simulink model "model_double_pendulum"  (R2021b)
settings: Solver=VariableStepAuto  StartTime=0.0  StopTime=10  RelTol=1e-3  EnableMultiTasking=on
InitFcn:
  | m=4;
  | m1=3;
  | m2=1.5;
  | l1=0.5;
  | l2=0.35;
  | g=9.81;
undefined symbols (not defined in the file or in its folder): A, A1_etm4, A1_zv, A2_etm4, A2_zv, A3_etm4, A4_etm4, B, b0, C, D1, Kd, Kp, L, l, L2, t2_etm4, t2_zv, t3_etm4, t4_etm4
settings Model: Creator=ADMIN  LastModifiedBy=Admin
settings DataIOCC: ReturnWorkspaceOutputs=off
settings OptimizationCC: LifeSpan=inf
settings DebuggingCC: SFUnexpectedBacktrackingDiag=warning  SFNoUnconditionalDefaultTransitionDiag=warning  SFMachineParentedDataDiag=warning  ArithmeticOperatorsInVariantConditions=warning
settings SFSimCC: SimUseLocalCustomCode=off  CustomCodeUndefinedFunction=UseInterfaceOnly
settings RTWCC: RTWUseLocalCustomCode=off
settings CodeAppCC: StateflowObjectComments=on
settings GRTTargetCC: TargetLangStandard=C89/C90 (ANSI)
settings ConfigComp: CovMetricSettings=dw  CovSaveCumulativeToWorkspaceVar=on  CovSaveSingleToWorkspaceVar=on  CovExternalEMLEnable=off

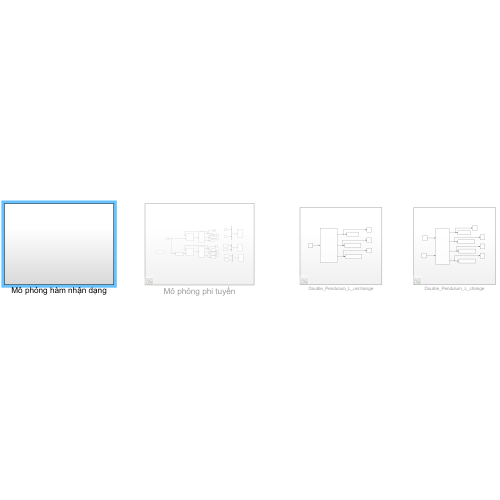
[thumbnail: Simulink's stored preview of the top-level diagram]
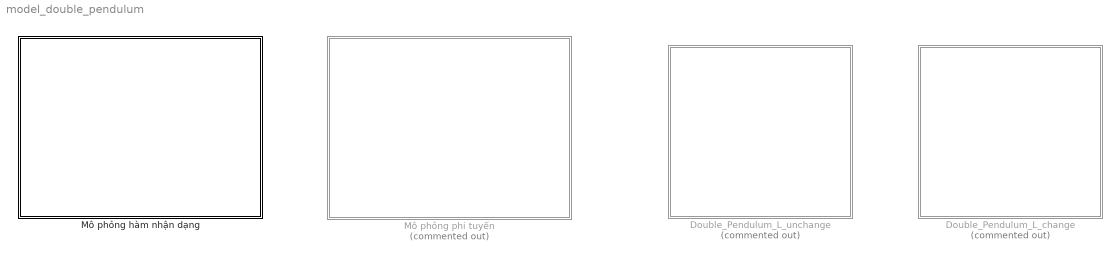
== system model_double_pendulum ==
  Double_Pendulum_L_change : Subsystem  Commented=on
  Double_Pendulum_L_unchange : Subsystem  Commented=on
  Mô phỏng hàm nhận dạng : Subsystem
  Mô phỏng phi tuyến : Subsystem  Commented=on

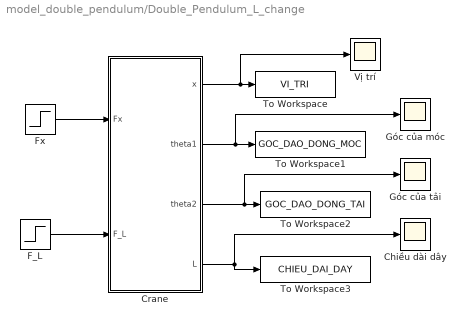
== system model_double_pendulum/Double_Pendulum_L_change ==
  Chiều dài dây : Scope
  "Crane " : Subsystem
  F_L : Step  Time=0  After=10  SampleTime=0
  Fx : Step  Time=0  After=10  SampleTime=0
  Góc của móc : Scope
  Góc của tải : Scope
  To Workspace : ToWorkspace  VariableName=VI_TRI  SaveFormat=Timeseries  SampleTime=-1
  To Workspace1 : ToWorkspace  VariableName=GOC_DAO_DONG_MOC  SaveFormat=Timeseries  SampleTime=-1
  To Workspace2 : ToWorkspace  VariableName=GOC_DAO_DONG_TAI  SaveFormat=Timeseries  SampleTime=-1
  To Workspace3 : ToWorkspace  VariableName=CHIEU_DAI_DAY  SaveFormat=Timeseries  SampleTime=-1
  Vị trí : Scope
  wires:
  Fx/1 -> "Crane "/1("Fx ")
  F_L/1 -> "Crane "/2(F_L)
  "Crane "/1("x ") -> Vị trí/1, To Workspace/1
  "Crane "/3(theta2) -> Góc của tải/1, To Workspace2/1
  "Crane "/4(L) -> To Workspace3/1, Chiều dài dây/1
  "Crane "/2(theta1) -> Góc của móc/1, To Workspace1/1

== system model_double_pendulum/Double_Pendulum_L_unchange ==
  "Crane " : Subsystem
  Fx : Step  Time=0  After=10  SampleTime=0
  Góc của móc : Scope
  Góc của tải : Scope
  To Workspace : ToWorkspace  VariableName=VI_TRI1  SaveFormat=Timeseries  SampleTime=-1
  To Workspace1 : ToWorkspace  VariableName=GOC_DAO_DONG_MOC1  SaveFormat=Timeseries  SampleTime=-1
  To Workspace2 : ToWorkspace  VariableName=GOC_DAO_DONG_TAI1  SaveFormat=Timeseries  SampleTime=-1
  Vị trí : Scope
  wires:
  "Crane "/2(theta1) -> Góc của móc/1, To Workspace1/1
  "Crane "/1("x ") -> Vị trí/1, To Workspace/1
  Fx/1 -> "Crane "/1("Fx ")
  "Crane "/3(theta2) -> Góc của tải/1, To Workspace2/1

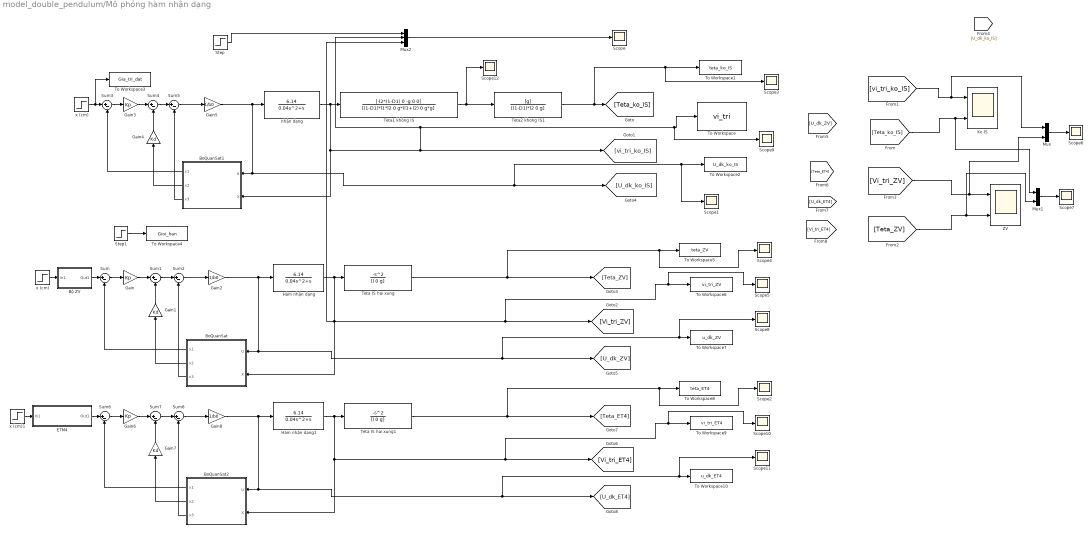
== system model_double_pendulum/Mô phỏng hàm nhận dạng ==
  " nhận dạng" : TransferFcn  Numerator=[6.14]  Denominator="[0.04 1  0]"
  BoQuanSat : Subsystem
  BoQuanSat1 : Subsystem
  BoQuanSat2 : Subsystem
  Bộ ZV : Subsystem
  ETM4 : Subsystem
  Gain : Gain  Gain=Kp
  Gain1 : Gain  Gain=Kd
  Gain2 : Gain  Gain=1/b0
  Gain3 : Gain  Gain=Kp
  Gain4 : Gain  Gain=Kd
  Gain5 : Gain  Gain=1/b0
  Gain6 : Gain  Gain=Kp
  Gain7 : Gain  Gain=Kd
  Gain8 : Gain  Gain=1/b0
  Hàm nhận dạng : TransferFcn  Numerator=[6.14]  Denominator="[0.04 1  0]"
  Hàm nhận dạng1 : TransferFcn  Numerator=[6.14]  Denominator="[0.04 1  0]"
  Ko IS : Scope  NumInputPorts=2
  Mux : Mux  Inputs=2
  Mux1 : Mux  Inputs=2
  Mux2 : Mux  Inputs=3
  Scope{,1..12} (13 alike) : Scope
  Step : Step  Time=0  After=49  SampleTime=0
  Step1 : Step  Time=0  After=10  SampleTime=0
  Sum{,1..8} (9 alike) : Sum  Inputs=|+-
  Teta IS hai xung : TransferFcn  Numerator=[-1 0 0]  Denominator=[l 0 g]
  Teta IS hai xung1 : TransferFcn  Numerator=[-1 0 0]  Denominator=[l 0 g]
  "Teta1 không IS " : TransferFcn  Numerator=[-l2*(1-D1) 0 -g 0 0]  Denominator=[(1-D1)*l1*l2 0 g*(l1+l2) 0 g*g]
  Teta2 khong IS1 : TransferFcn  Numerator=[g]  Denominator=[(1-D1)*l2 0 g]
  To Workspace : ToWorkspace  VariableName=vi_tri  SaveFormat=Timeseries  SampleTime=0.005
  To Workspace1 : ToWorkspace  VariableName=teta_ko_IS  SaveFormat=Timeseries  SampleTime=-1
  To Workspace10 : ToWorkspace  VariableName=u_dk_ET4  SaveFormat=Timeseries  SampleTime=-1
  To Workspace2 : ToWorkspace  VariableName=U_dk_ko_IS  SaveFormat=Timeseries  SampleTime=-1
  To Workspace3 : ToWorkspace  VariableName=Gia_tri_dat  SaveFormat=Timeseries  SampleTime=0.005
  To Workspace4 : ToWorkspace  VariableName=Gioi_han  SaveFormat=Timeseries  SampleTime=-1
  To Workspace5 : ToWorkspace  VariableName=teta_ZV  SaveFormat=Timeseries  SampleTime=-1
  To Workspace6 : ToWorkspace  VariableName=vi_tri_ZV  SaveFormat=Timeseries  SampleTime=-1
  To Workspace7 : ToWorkspace  VariableName=u_dk_ZV  SaveFormat=Timeseries  SampleTime=-1
  To Workspace8 : ToWorkspace  VariableName=teta_ET4  SaveFormat=Timeseries  SampleTime=-1
  To Workspace9 : ToWorkspace  VariableName=vi_tri_ET4  SaveFormat=Timeseries  SampleTime=-1
  ZV : Scope  NumInputPorts=2
  x (cm) : Step  Time=0  After=50  SampleTime=0
  "x (cm) " : Step  Time=0  After=50  SampleTime=0
  x (cm)1 : Step  Time=0  After=50  SampleTime=0
  wires:
  Gain/1 -> Sum1/1
  Sum2/1 -> Gain2/1
  BoQuanSat/2(x2) -> Gain1/1
  BoQuanSat/3(x3) -> Sum2/2
  BoQuanSat/1(x1) -> Sum/2
  Sum/1 -> Gain/1
  Sum1/1 -> Sum2/1
  Gain1/1 -> Sum1/2
  Gain2/1 -> Hàm nhận dạng/1, Scope8/1, To Workspace7/1, [U_dk_ZV], BoQuanSat/1(U)
  x (cm)/1 -> Bộ ZV/1(In1)
  Bộ ZV/1(Out1) -> Sum/1
  Gain4/1 -> Sum4/2
  Sum4/1 -> Sum5/1
  Sum5/1 -> Gain5/1
  BoQuanSat1/1(x1) -> Sum3/2
  BoQuanSat1/3(x3) -> Sum5/2
  BoQuanSat1/2(x2) -> Gain4/1
  Sum3/1 -> Gain3/1
  Gain3/1 -> Sum4/1
  Teta IS hai xung/1 -> Scope4/1, To Workspace5/1, [Teta_ZV]
  [vi_tri_ko_IS] -> Mux/1, Ko IS/1
  [Vi_tri_ZV] -> Mux/2, ZV/1
  [Teta_ZV] -> Mux1/2, ZV/2
  [Teta_ko_IS] -> Mux1/1, Ko IS/2
  Mux/1 -> Scope6/1
  Mux1/1 -> Scope7/1
  " nhận dạng"/1 -> "Teta1 không IS "/1, Scope9/1, To Workspace/1, Mux2/2, [vi_tri_ko_IS], BoQuanSat1/2(X)
  Gain5/1 -> " nhận dạng"/1, Scope1/1, To Workspace2/1, [U_dk_ko_IS], BoQuanSat1/1(U)
  Hàm nhận dạng/1 -> Teta IS hai xung/1, Scope5/1, To Workspace6/1, [Vi_tri_ZV], Mux2/3, BoQuanSat/2(X)
  Step/1 -> Mux2/1
  Mux2/1 -> Scope/1
  "x (cm) "/1 -> To Workspace3/1, Sum3/1
  Step1/1 -> To Workspace4/1
  BoQuanSat2/3(x3) -> Sum8/2
  Teta IS hai xung1/1 -> Scope2/1, To Workspace8/1, [Teta_ET4]
  x (cm)1/1 -> ETM4/1(In1)
  ETM4/1(Out1) -> Sum6/1
  Hàm nhận dạng1/1 -> Teta IS hai xung1/1, Scope10/1, To Workspace9/1, [Vi_tri_ET4], BoQuanSat2/2(X)
  BoQuanSat2/2(x2) -> Gain7/1
  Sum7/1 -> Sum8/1
  BoQuanSat2/1(x1) -> Sum6/2
  Sum6/1 -> Gain6/1
  Sum8/1 -> Gain8/1
  Gain6/1 -> Sum7/1
  Gain8/1 -> Hàm nhận dạng1/1, Scope11/1, To Workspace10/1, [U_dk_ET4], BoQuanSat2/1(U)
  Gain7/1 -> Sum7/2
  "Teta1 không IS "/1 -> Teta2 khong IS1/1, Scope12/1
  Teta2 khong IS1/1 -> Scope3/1, To Workspace1/1, [Teta_ko_IS]

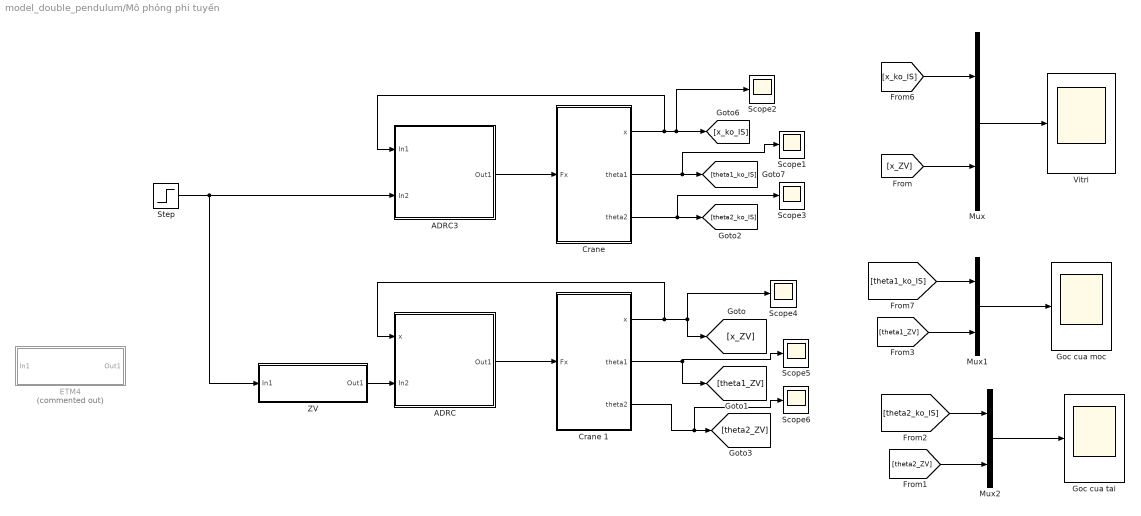
== system model_double_pendulum/Mô phỏng phi tuyến ==
  ADRC : Subsystem
  ADRC3 : Subsystem
  "Crane " : Subsystem
  Crane 1 : Subsystem
  ETM4 : Subsystem  Commented=on
  Goc cua moc : Scope
  Goc cua tai : Scope
  Mux : Mux  Inputs=2
  Mux1 : Mux  Inputs=2
  Mux2 : Mux  Inputs=2
  Scope{1..6} (6 alike) : Scope
  Step : Step  Time=0  After=40  SampleTime=0
  Vitri : Scope
  ZV : Subsystem
  wires:
  [theta1_ko_IS] -> Mux1/1
  Crane 1/1("x ") -> [x_ZV], Scope4/1, ADRC/1("x ")
  Mux1/1 -> Goc cua moc/1
  ADRC/1(Out1) -> Crane 1/1("Fx ")
  Step/1 -> ADRC3/2(In2), ZV/1(In1)
  Mux/1 -> Vitri/1
  [x_ko_IS] -> Mux/1
  "Crane "/1("x ") -> Scope2/1, [x_ko_IS], ADRC3/1(In1)
  ADRC3/1(Out1) -> "Crane "/1("Fx ")
  "Crane "/2(theta1) -> Scope1/1, [theta1_ko_IS]
  ZV/1(Out1) -> ADRC/2(In2)
  [x_ZV] -> Mux/2
  "Crane "/3(theta2) -> Scope3/1, [theta2_ko_IS]
  Crane 1/2(theta1) -> [theta1_ZV], Scope5/1
  [theta1_ZV] -> Mux1/2
  Crane 1/3(theta2) -> Scope6/1, [theta2_ZV]
  [theta2_ZV] -> Mux2/2
  Mux2/1 -> Goc cua tai/1
  [theta2_ko_IS] -> Mux2/1

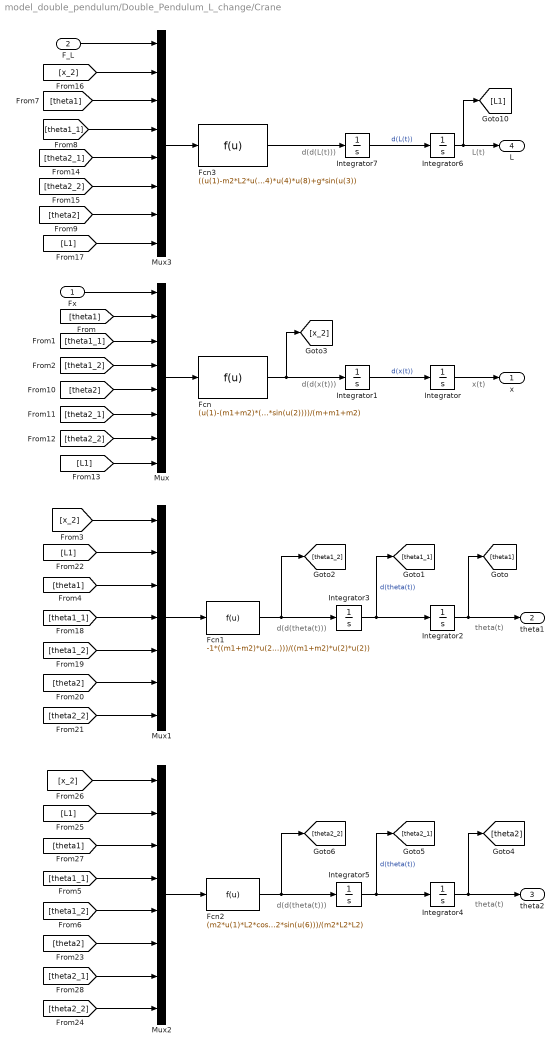
== system model_double_pendulum/Double_Pendulum_L_change/Crane  ==
  note: d(d(x(t)))
  note: x(t)
  note: d(d(theta(t)))
  note: theta(t)
  note: d(d(theta(t)))
  note: theta(t)
  note: L(t)
  note: d(d(L(t)))
  "Fx " : Inport
  F_L : Inport  Port=2
  Fcn : Fcn  Expr=(u(1)-(m1+m2)*(u(4)*u(8)*cos(u(2))-u(3)*u(3)*u(8)*sin(u(2))))/(m+m1+m2)
  Fcn1 : Fcn  Expr=-1*((m1+m2)*u(2)*u(1)*cos(u(3))+m2*u(2)*L2*(u(7)*cos(u(3)-u(6))+u(4)*u(4)*sin(u(3)-u(6)))+(m1+m2)*g*u(2)*sin(u(3)))/((m1+m2)*u(2)*u(2))
  Fcn2 : Fcn  Expr=(m2*u(1)*L2*cos(u(6))+m2*u(2)*L2*u(5)*cos(u(3)-u(6))-m2*u(2)*L2*u(4)*u(4)*sin(u(3)-u(6))+m2*g*L2*sin(u(6)))/(m2*L2*L2)
  Fcn3 : Fcn  Expr=((u(1)-m2*L2*u(6)*sin(u(3)-u(7))+m2*L2*u(5)*u(5)*cos(u(3)-u(7)))/(m1+m2))-u(2)*sin(u(3))+u(4)*u(4)*u(8)+g*sin(u(3))
  Integrator{,1..5,7} (7 alike) : Integrator
  Integrator6 : Integrator  InitialCondition=0.5
  Mux : Mux  Inputs=8
  Mux1 : Mux  Inputs=7
  Mux2 : Mux  Inputs=8
  Mux3 : Mux  Inputs=8
  "x " : Outport
  theta1 : Outport  Port=2
  theta2 : Outport  Port=3
  L : Outport  Port=4
  wires:
  Integrator/1 -> "x "/1
  Integrator1/1 -> Integrator/1  "d(x(t))"
  Integrator2/1 -> [theta1], theta1/1
  Integrator3/1 -> [theta1_1], Integrator2/1  "d(theta(t))"
  Fcn/1 -> [x_2], Integrator1/1
  Mux/1 -> Fcn/1
  "Fx "/1 -> Mux/1
  [theta1] -> Mux/2
  [theta1_1] -> Mux/3
  [theta1_2] -> Mux/4
  Mux1/1 -> Fcn1/1
  Fcn1/1 -> [theta1_2], Integrator3/1
  Mux2/1 -> Fcn2/1
  Fcn2/1 -> [theta2_2], Integrator5/1
  Integrator5/1 -> [theta2_1], Integrator4/1  "d(theta(t))"
  Integrator4/1 -> [theta2], theta2/1
  F_L/1 -> Mux3/1
  Mux3/1 -> Fcn3/1
  Fcn3/1 -> Integrator7/1
  Integrator7/1 -> Integrator6/1  "d(L(t))"
  Integrator6/1 -> [L1], L/1
  [theta2] -> Mux/5
  [theta2_1] -> Mux/6
  [theta2_2] -> Mux/7
  [L1] -> Mux/8
  [theta2_1] -> Mux3/5
  [theta2_2] -> Mux3/6
  [theta1] -> Mux3/3
  [theta1_1] -> Mux3/4
  [x_2] -> Mux3/2
  [theta2] -> Mux3/7
  [L1] -> Mux3/8
  [x_2] -> Mux1/1
  [L1] -> Mux1/2
  [theta1] -> Mux1/3
  [theta1_1] -> Mux1/4
  [theta1_2] -> Mux1/5
  [theta2] -> Mux1/6
  [theta2_2] -> Mux1/7
  [x_2] -> Mux2/1
  [L1] -> Mux2/2
  [theta1] -> Mux2/3
  [theta1_1] -> Mux2/4
  [theta1_2] -> Mux2/5
  [theta2] -> Mux2/6
  [theta2_1] -> Mux2/7
  [theta2_2] -> Mux2/8

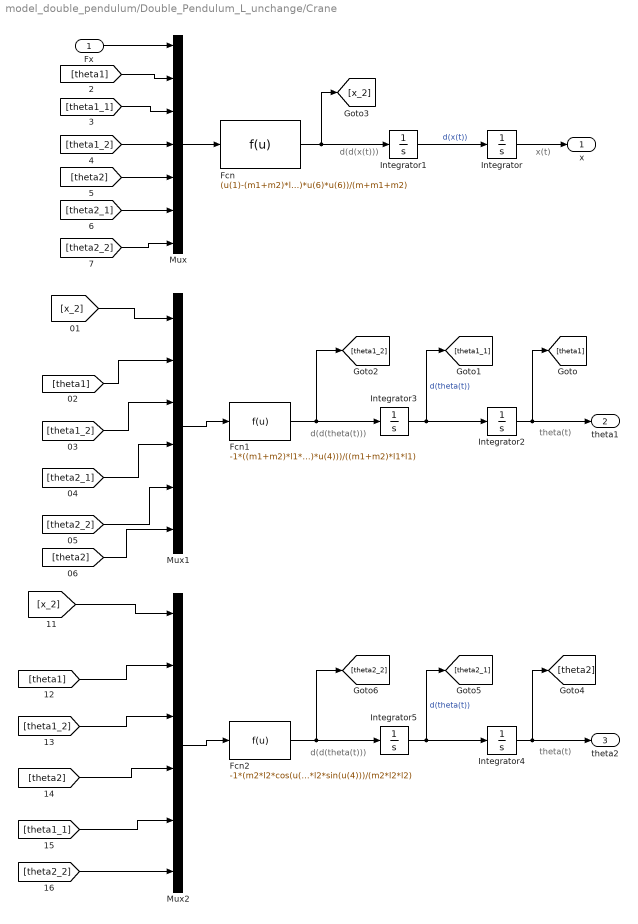
== system model_double_pendulum/Double_Pendulum_L_unchange/Crane  ==
  note: d(d(x(t)))
  note: x(t)
  note: d(d(theta(t)))
  note: theta(t)
  note: d(d(theta(t)))
  note: theta(t)
  "Fx " : Inport
  Fcn : Fcn  Expr=(u(1)-(m1+m2)*l1*(cos(u(2))*u(4)-sin(u(2))*u(3)*u(3))-m2*l2*u(7)*cos(u(5))+m2*l2*sin(u(5))*u(6)*u(6))/(m+m1+m2)
  Fcn1 : Fcn  Expr=-1*((m1+m2)*l1*u(1)*cos(u(2))+(m1+m2)*(g*l1*sin(u(2))+l1*l1*u(3))+m2*l1*l2*(cos(u(2)-u(6))*u(5)+sin(u(2)-u(6))*u(4)*u(4)))/((m1+m2)*l1*l1)
  Fcn2 : Fcn  Expr=-1*(m2*l2*cos(u(4))*u(1)+m2*l1*l2*cos(u(2)-u(4))*u(3)-m2*l1*l2*sin(u(2)-u(4))*u(5)*u(5)+m2*g*l2*sin(u(4)))/(m2*l2*l2)
  Integrator{,1..5} (6 alike) : Integrator
  Mux : Mux  Inputs=7
  Mux1 : Mux  Inputs=6
  Mux2 : Mux  Inputs=6
  "x " : Outport
  theta1 : Outport  Port=2
  theta2 : Outport  Port=3
  wires:
  Integrator/1 -> "x "/1
  Integrator1/1 -> Integrator/1  "d(x(t))"
  Integrator2/1 -> [theta1], theta1/1
  Integrator3/1 -> [theta1_1], Integrator2/1  "d(theta(t))"
  Fcn/1 -> [x_2], Integrator1/1
  Mux/1 -> Fcn/1
  "Fx "/1 -> Mux/1
  [theta1] -> Mux/2
  [theta1_1] -> Mux/3
  [theta1_2] -> Mux/4
  Mux1/1 -> Fcn1/1
  Fcn1/1 -> [theta1_2], Integrator3/1
  Mux2/1 -> Fcn2/1
  Fcn2/1 -> [theta2_2], Integrator5/1
  Integrator5/1 -> [theta2_1], Integrator4/1  "d(theta(t))"
  Integrator4/1 -> [theta2], theta2/1
  [theta2] -> Mux/5
  [theta2_1] -> Mux/6
  [theta2_2] -> Mux/7
  [x_2] -> Mux1/1
  [theta1] -> Mux1/2
  [theta2_2] -> Mux1/5
  [theta2_1] -> Mux1/4
  [theta1_2] -> Mux1/3
  [theta2] -> Mux1/6
  [x_2] -> Mux2/1
  [theta2] -> Mux2/4
  [theta2_2] -> Mux2/6
  [theta1] -> Mux2/2
  [theta1_1] -> Mux2/5
  [theta1_2] -> Mux2/3

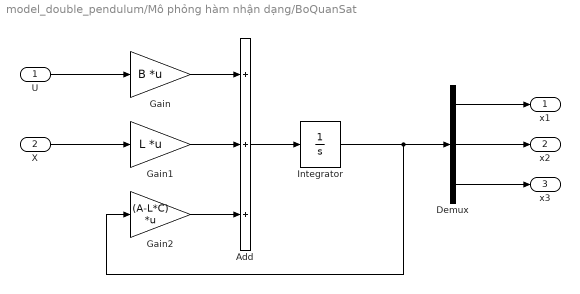
== system model_double_pendulum/Mô phỏng hàm nhận dạng/BoQuanSat ==
  U : Inport
  X : Inport  Port=2
  Add : Sum  Inputs=+++
  Demux : Demux  Outputs=3
  Gain : Gain  Gain=B  Multiplication=Matrix(K*u)
  Gain1 : Gain  Gain=L  Multiplication=Matrix(K*u)
  Gain2 : Gain  Gain=(A-L*C)  Multiplication=Matrix(K*u)
  Integrator : Integrator
  x1 : Outport
  x2 : Outport  Port=2
  x3 : Outport  Port=3
  wires:
  Demux/1 -> x1/1
  Add/1 -> Integrator/1
  Integrator/1 -> Demux/1, Gain2/1
  U/1 -> Gain/1
  Demux/3 -> x3/1
  Gain1/1 -> Add/2
  Gain2/1 -> Add/3
  X/1 -> Gain1/1
  Gain/1 -> Add/1
  Demux/2 -> x2/1

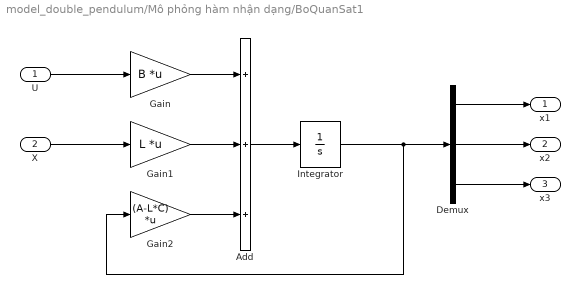
== system model_double_pendulum/Mô phỏng hàm nhận dạng/BoQuanSat1 ==
  U : Inport
  X : Inport  Port=2
  Add : Sum  Inputs=+++
  Demux : Demux  Outputs=3
  Gain : Gain  Gain=B  Multiplication=Matrix(K*u)
  Gain1 : Gain  Gain=L  Multiplication=Matrix(K*u)
  Gain2 : Gain  Gain=(A-L*C)  Multiplication=Matrix(K*u)
  Integrator : Integrator
  x1 : Outport
  x2 : Outport  Port=2
  x3 : Outport  Port=3
  wires:
  Demux/1 -> x1/1
  Add/1 -> Integrator/1
  Integrator/1 -> Demux/1, Gain2/1
  U/1 -> Gain/1
  Demux/3 -> x3/1
  Gain1/1 -> Add/2
  Gain2/1 -> Add/3
  X/1 -> Gain1/1
  Gain/1 -> Add/1
  Demux/2 -> x2/1

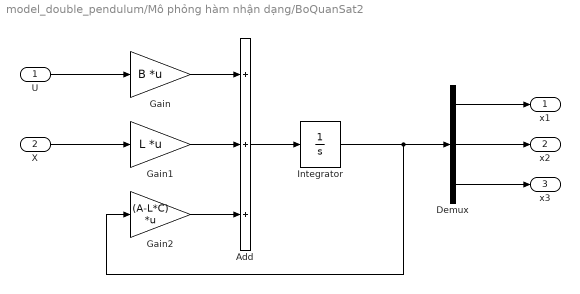
== system model_double_pendulum/Mô phỏng hàm nhận dạng/BoQuanSat2 ==
  U : Inport
  X : Inport  Port=2
  Add : Sum  Inputs=+++
  Demux : Demux  Outputs=3
  Gain : Gain  Gain=B  Multiplication=Matrix(K*u)
  Gain1 : Gain  Gain=L  Multiplication=Matrix(K*u)
  Gain2 : Gain  Gain=(A-L*C)  Multiplication=Matrix(K*u)
  Integrator : Integrator
  x1 : Outport
  x2 : Outport  Port=2
  x3 : Outport  Port=3
  wires:
  Demux/1 -> x1/1
  Add/1 -> Integrator/1
  Integrator/1 -> Demux/1, Gain2/1
  U/1 -> Gain/1
  Demux/3 -> x3/1
  Gain1/1 -> Add/2
  Gain2/1 -> Add/3
  X/1 -> Gain1/1
  Gain/1 -> Add/1
  Demux/2 -> x2/1

== system model_double_pendulum/Mô phỏng hàm nhận dạng/Bộ ZV ==
  In1 : Inport
  Gain : Gain  Gain=A1_zv
  Gain1 : Gain  Gain=A2_zv
  Sum : Sum  Inputs=|++
  Transport Delay : TransportDelay  DelayTime=t2_zv
  Out1 : Outport
  wires:
  In1/1 -> Gain1/1, Gain/1
  Gain/1 -> Sum/1
  Gain1/1 -> Transport Delay/1
  Transport Delay/1 -> Sum/2
  Sum/1 -> Out1/1

== system model_double_pendulum/Mô phỏng hàm nhận dạng/ETM4 ==
  In1 : Inport
  Gain : Gain  Gain=A1_etm4
  Gain1 : Gain  Gain=A2_etm4
  Gain2 : Gain  Gain=A3_etm4
  Gain3 : Gain  Gain=A4_etm4
  Sum : Sum  Inputs=++++
  Transport Delay : TransportDelay  DelayTime=t2_etm4
  Transport Delay1 : TransportDelay  DelayTime=t3_etm4
  Transport Delay2 : TransportDelay  DelayTime=t4_etm4
  Out1 : Outport
  wires:
  In1/1 -> Gain1/1, Gain3/1, Gain2/1, Gain/1
  Gain1/1 -> Transport Delay/1
  Transport Delay/1 -> Sum/2
  Sum/1 -> Out1/1
  Gain2/1 -> Transport Delay1/1
  Gain/1 -> Sum/1
  Transport Delay1/1 -> Sum/3
  Gain3/1 -> Transport Delay2/1
  Transport Delay2/1 -> Sum/4

== system model_double_pendulum/Mô phỏng phi tuyến/ADRC ==
  "x " : Inport
  In2 : Inport  Port=2
  BoQuanSat : Subsystem
  Gain : Gain  Gain=Kp
  Gain1 : Gain  Gain=Kd
  Gain2 : Gain  Gain=1/b0
  Sum : Sum  Inputs=|+-
  Sum1 : Sum  Inputs=|+-
  Sum2 : Sum  Inputs=|+-
  Out1 : Outport
  wires:
  Gain/1 -> Sum1/1
  Sum2/1 -> Gain2/1
  In2/1 -> Sum/1
  BoQuanSat/2(x2) -> Gain1/1
  BoQuanSat/3(x3) -> Sum2/2
  BoQuanSat/1(x1) -> Sum/2
  Sum/1 -> Gain/1
  Sum1/1 -> Sum2/1
  Gain1/1 -> Sum1/2
  Gain2/1 -> Out1/1, BoQuanSat/1(U(t))
  "x "/1 -> BoQuanSat/2(Y(t))

== system model_double_pendulum/Mô phỏng phi tuyến/ADRC3 ==
  In1 : Inport
  In2 : Inport  Port=2
  BoQuanSat : Subsystem
  Gain : Gain  Gain=Kp
  Gain1 : Gain  Gain=Kd
  Gain2 : Gain  Gain=1/b0
  Sum : Sum  Inputs=|+-
  Sum1 : Sum  Inputs=|+-
  Sum2 : Sum  Inputs=|+-
  Out1 : Outport
  wires:
  Gain/1 -> Sum1/1
  Sum2/1 -> Gain2/1
  In2/1 -> Sum/1
  BoQuanSat/2(x2) -> Gain1/1
  BoQuanSat/3(x3) -> Sum2/2
  BoQuanSat/1(x1) -> Sum/2
  Sum/1 -> Gain/1
  Sum1/1 -> Sum2/1
  Gain1/1 -> Sum1/2
  Gain2/1 -> Out1/1, BoQuanSat/1(U(t))
  In1/1 -> BoQuanSat/2(Y(t))

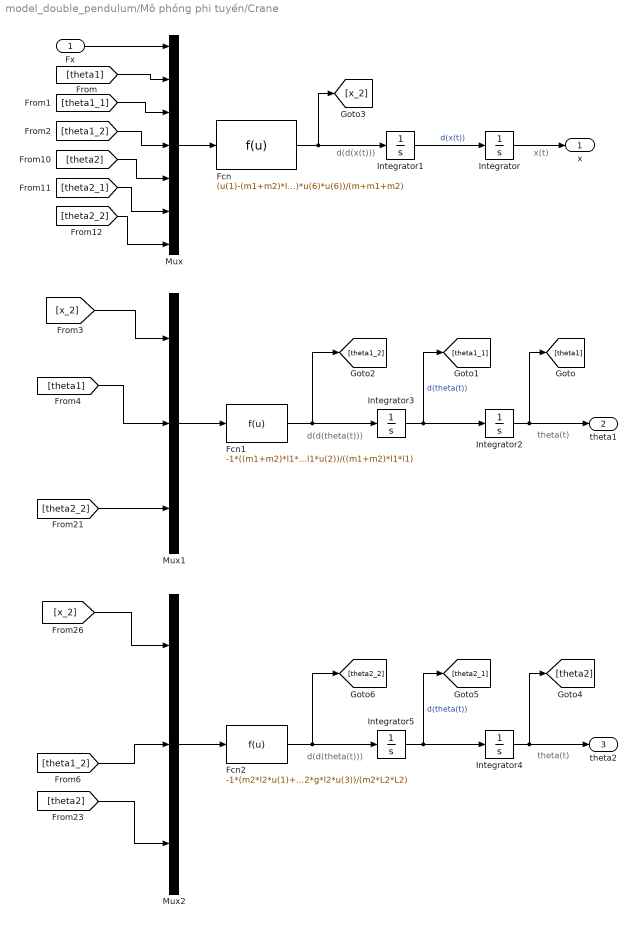
== system model_double_pendulum/Mô phỏng phi tuyến/Crane  ==
  note: d(d(x(t)))
  note: x(t)
  note: d(d(theta(t)))
  note: theta(t)
  note: d(d(theta(t)))
  note: theta(t)
  "Fx " : Inport
  Fcn : Fcn  Expr=(u(1)-(m1+m2)*l1*(u(4)-u(2)*u(3)*u(3))+m2*l2*u(7)-m2*l2*u(5)*u(6)*u(6))/(m+m1+m2)
  Fcn1 : Fcn  Expr=-1*((m1+m2)*l1*u(1)+m2*l1*l2*u(3)+(m1+m2)*g*l1*u(2))/((m1+m2)*l1*l1)
  Fcn2 : Fcn  Expr=-1*(m2*l2*u(1)+m2*l1*l2*u(2)+m2*g*l2*u(3))/(m2*L2*L2)
  Integrator{,1..5} (6 alike) : Integrator
  Mux : Mux  Inputs=7
  Mux1 : Mux  Inputs=3
  Mux2 : Mux  Inputs=3
  "x " : Outport
  theta1 : Outport  Port=2
  theta2 : Outport  Port=3
  wires:
  Integrator/1 -> "x "/1
  Integrator1/1 -> Integrator/1  "d(x(t))"
  Integrator2/1 -> [theta1], theta1/1
  Integrator3/1 -> [theta1_1], Integrator2/1  "d(theta(t))"
  Fcn/1 -> [x_2], Integrator1/1
  Mux/1 -> Fcn/1
  "Fx "/1 -> Mux/1
  [theta1] -> Mux/2
  [theta1_1] -> Mux/3
  [theta1_2] -> Mux/4
  Mux1/1 -> Fcn1/1
  Fcn1/1 -> [theta1_2], Integrator3/1
  Mux2/1 -> Fcn2/1
  Fcn2/1 -> [theta2_2], Integrator5/1
  Integrator5/1 -> [theta2_1], Integrator4/1  "d(theta(t))"
  Integrator4/1 -> [theta2], theta2/1
  [theta2] -> Mux/5
  [theta2_1] -> Mux/6
  [theta2_2] -> Mux/7
  [x_2] -> Mux1/1
  [x_2] -> Mux2/1
  [theta1] -> Mux1/2
  [theta2_2] -> Mux1/3
  [theta1_2] -> Mux2/2
  [theta2] -> Mux2/3

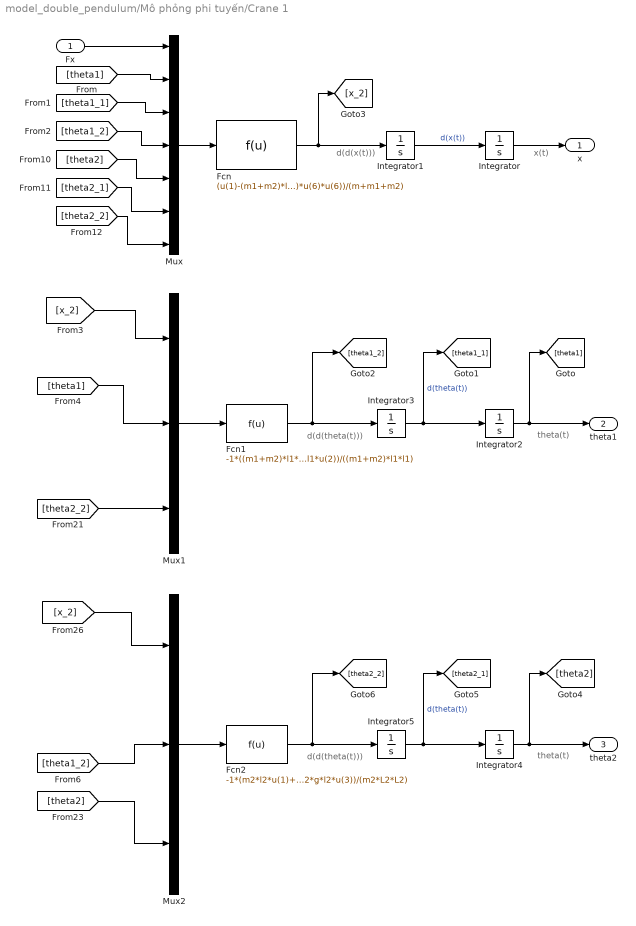
== system model_double_pendulum/Mô phỏng phi tuyến/Crane 1 ==
  note: d(d(x(t)))
  note: x(t)
  note: d(d(theta(t)))
  note: theta(t)
  note: d(d(theta(t)))
  note: theta(t)
  "Fx " : Inport
  Fcn : Fcn  Expr=(u(1)-(m1+m2)*l1*(u(4)-u(2)*u(3)*u(3))+m2*l2*u(7)-m2*l2*u(5)*u(6)*u(6))/(m+m1+m2)
  Fcn1 : Fcn  Expr=-1*((m1+m2)*l1*u(1)+m2*l1*l2*u(3)+(m1+m2)*g*l1*u(2))/((m1+m2)*l1*l1)
  Fcn2 : Fcn  Expr=-1*(m2*l2*u(1)+m2*l1*l2*u(2)+m2*g*l2*u(3))/(m2*L2*L2)
  Integrator{,1..5} (6 alike) : Integrator
  Mux : Mux  Inputs=7
  Mux1 : Mux  Inputs=3
  Mux2 : Mux  Inputs=3
  "x " : Outport
  theta1 : Outport  Port=2
  theta2 : Outport  Port=3
  wires:
  Integrator/1 -> "x "/1
  Integrator1/1 -> Integrator/1  "d(x(t))"
  Integrator2/1 -> [theta1], theta1/1
  Integrator3/1 -> [theta1_1], Integrator2/1  "d(theta(t))"
  Fcn/1 -> [x_2], Integrator1/1
  Mux/1 -> Fcn/1
  "Fx "/1 -> Mux/1
  [theta1] -> Mux/2
  [theta1_1] -> Mux/3
  [theta1_2] -> Mux/4
  Mux1/1 -> Fcn1/1
  Fcn1/1 -> [theta1_2], Integrator3/1
  Mux2/1 -> Fcn2/1
  Fcn2/1 -> [theta2_2], Integrator5/1
  Integrator5/1 -> [theta2_1], Integrator4/1  "d(theta(t))"
  Integrator4/1 -> [theta2], theta2/1
  [theta2] -> Mux/5
  [theta2_1] -> Mux/6
  [theta2_2] -> Mux/7
  [x_2] -> Mux1/1
  [x_2] -> Mux2/1
  [theta1] -> Mux1/2
  [theta2_2] -> Mux1/3
  [theta1_2] -> Mux2/2
  [theta2] -> Mux2/3

== system model_double_pendulum/Mô phỏng phi tuyến/ETM4 ==
  In1 : Inport
  Gain : Gain  Gain=A1_etm4
  Gain1 : Gain  Gain=A2_etm4
  Gain2 : Gain  Gain=A3_etm4
  Gain3 : Gain  Gain=A4_etm4
  Sum : Sum  Inputs=++++
  Transport Delay : TransportDelay  DelayTime=t2_etm4
  Transport Delay1 : TransportDelay  DelayTime=t3_etm4
  Transport Delay2 : TransportDelay  DelayTime=t4_etm4
  Out1 : Outport
  wires:
  In1/1 -> Gain1/1, Gain3/1, Gain2/1, Gain/1
  Gain1/1 -> Transport Delay/1
  Transport Delay/1 -> Sum/2
  Sum/1 -> Out1/1
  Gain2/1 -> Transport Delay1/1
  Gain/1 -> Sum/1
  Transport Delay1/1 -> Sum/3
  Gain3/1 -> Transport Delay2/1
  Transport Delay2/1 -> Sum/4

== system model_double_pendulum/Mô phỏng phi tuyến/ZV ==
  In1 : Inport
  Gain : Gain  Gain=A1_zv
  Gain1 : Gain  Gain=A2_zv
  Sum : Sum  Inputs=|++
  Transport Delay : TransportDelay  DelayTime=t2_zv
  Out1 : Outport
  wires:
  In1/1 -> Gain1/1, Gain/1
  Gain/1 -> Sum/1
  Gain1/1 -> Transport Delay/1
  Transport Delay/1 -> Sum/2
  Sum/1 -> Out1/1

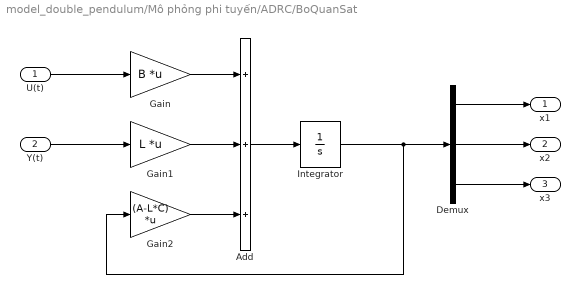
== system model_double_pendulum/Mô phỏng phi tuyến/ADRC/BoQuanSat ==
  U(t) : Inport
  Y(t) : Inport  Port=2
  Add : Sum  Inputs=+++
  Demux : Demux  Outputs=3
  Gain : Gain  Gain=B  Multiplication=Matrix(K*u)
  Gain1 : Gain  Gain=L  Multiplication=Matrix(K*u)
  Gain2 : Gain  Gain=(A-L*C)  Multiplication=Matrix(K*u)
  Integrator : Integrator
  x1 : Outport
  x2 : Outport  Port=2
  x3 : Outport  Port=3
  wires:
  Demux/1 -> x1/1
  Add/1 -> Integrator/1
  Integrator/1 -> Demux/1, Gain2/1
  U(t)/1 -> Gain/1
  Demux/3 -> x3/1
  Gain1/1 -> Add/2
  Gain2/1 -> Add/3
  Y(t)/1 -> Gain1/1
  Gain/1 -> Add/1
  Demux/2 -> x2/1

== system model_double_pendulum/Mô phỏng phi tuyến/ADRC3/BoQuanSat ==
  U(t) : Inport
  Y(t) : Inport  Port=2
  Add : Sum  Inputs=+++
  Demux : Demux  Outputs=3
  Gain : Gain  Gain=B  Multiplication=Matrix(K*u)
  Gain1 : Gain  Gain=L  Multiplication=Matrix(K*u)
  Gain2 : Gain  Gain=(A-L*C)  Multiplication=Matrix(K*u)
  Integrator : Integrator
  x1 : Outport
  x2 : Outport  Port=2
  x3 : Outport  Port=3
  wires:
  Demux/1 -> x1/1
  Add/1 -> Integrator/1
  Integrator/1 -> Demux/1, Gain2/1
  U(t)/1 -> Gain/1
  Demux/3 -> x3/1
  Gain1/1 -> Add/2
  Gain2/1 -> Add/3
  Y(t)/1 -> Gain1/1
  Gain/1 -> Add/1
  Demux/2 -> x2/1
